simulink model "LotkiVoltera"  (R2021b)
settings: Solver=VariableStepAuto  StartTime=0.0  StopTime=20  RelTol=1e-3
settings Model: Creator=Tymon  LastModifiedBy=Tymon

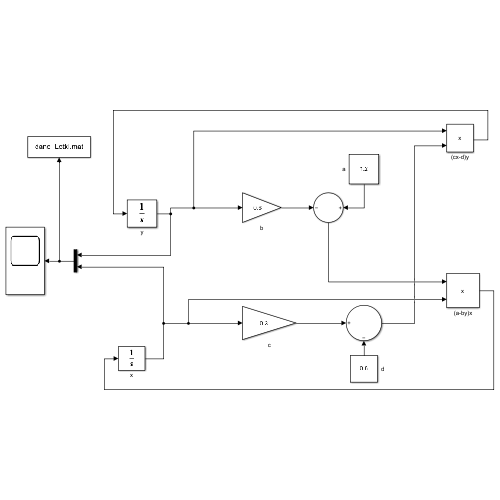
[thumbnail: Simulink's stored preview of the top-level diagram]
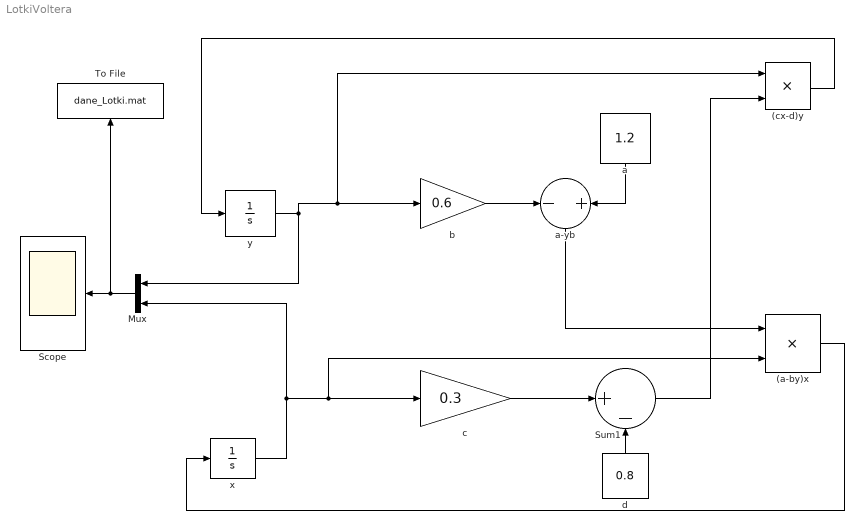
== system LotkiVoltera ==
  (a-by)x : Product
  (cx-d)y : Product
  Mux : Mux  Inputs=2
  Scope : Scope
  Sum1 : Sum  Inputs=|+-
  To File : ToFile  Filename=dane_Lotki.mat
  a : Constant  Value=1.2
  a-yb : Sum  Inputs=-+
  b : Gain  Gain=0.6
  c : Gain  Gain=0.3
  d : Constant  Value=0.8
  x : Integrator  InitialCondition=1
  y : Integrator  InitialCondition=2
  wires:
  x/1 -> Mux/2, (a-by)x/2, c/1
  y/1 -> (cx-d)y/1, b/1, Mux/1
  c/1 -> Sum1/1
  d/1 -> Sum1/2
  a/1 -> a-yb/2
  b/1 -> a-yb/1
  Sum1/1 -> (cx-d)y/2
  a-yb/1 -> (a-by)x/1
  (cx-d)y/1 -> y/1
  (a-by)x/1 -> x/1
  Mux/1 -> To File/1, Scope/1
